simulink model "sim_real_data"  (R2022b)
settings: Solver=FixedStepAuto  StartTime=0.0  StopTime=15  FixedStep=0.002  RelTol=1e-3
undefined symbols (not defined in the file): c, c0, dT, k, k0
libraries: sharedTrackingLibrary x2, simulink x1
settings Model: Creator=lucabeber  LastModifiedBy=lucabeber

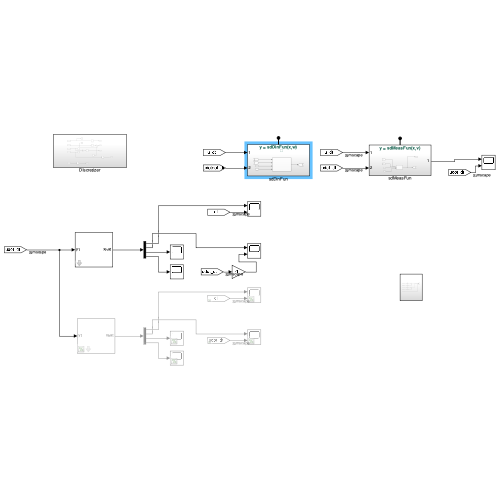
[thumbnail: Simulink's stored preview of the top-level diagram]
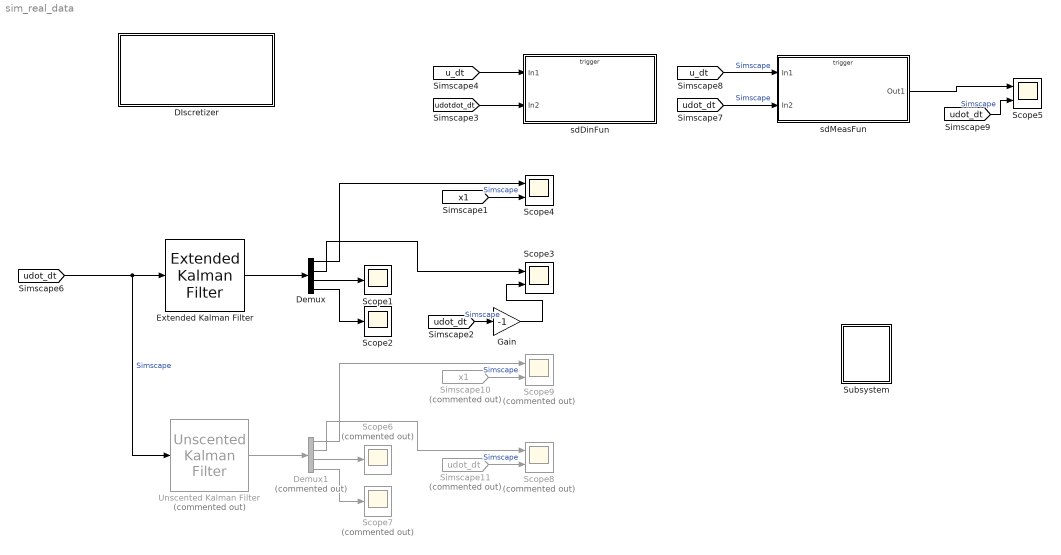
== system sim_real_data ==
  DIscretizer : Subsystem
  Demux : Demux
  Demux1 : Demux  Commented=on
  Extended Kalman Filter : sharedTrackingLibrary/Extended Kalman Filter  StateTransitionFcn=sdDinFun  HasStateTransitionJacobianFcn=off  HasAdditiveProcessNoise=Nonadditive  ProcessNoise=0  HasTimeVaryingProcessNoise=off  HasStateTransitionFcnExtraArgument=0  InitialState=[0,0,5e4,50]  InitialStateCovariance=[1,1,1e7,10]  MeasurementFcn1=sdMeasFun  HasMeasurementJacobianFcn1=off  HasMeasurementEnablePort1=off  HasAdditiveMeasurementNoise1=Nonadditive  MeasurementNoise1=0.00005  HasTimeVaryingMeasurementNoise1=off  HasMeasurementFcnExtraArgument1=0  HasMeasurementWrapping1=off  MeasurementFcn2=myMeasurementFcn  HasMeasurementJacobianFcn2=off  HasMeasurementEnablePort2=off  HasAdditiveMeasurementNoise2=Additive  MeasurementNoise2=1  HasTimeVaryingMeasurementNoise2=off  HasMeasurementFcnExtraArgument2=0  HasMeasurementWrapping2=off  MeasurementFcn3=myMeasurementFcn  HasMeasurementJacobianFcn3=off  HasMeasurementEnablePort3=off  HasAdditiveMeasurementNoise3=Additive  MeasurementNoise3=1  HasTimeVaryingMeasurementNoise3=off  HasMeasurementFcnExtraArgument3=0  HasMeasurementWrapping3=off  MeasurementFcn4=myMeasurementFcn  HasMeasurementJacobianFcn4=off  HasMeasurementEnablePort4=off  HasAdditiveMeasurementNoise4=Additive  MeasurementNoise4=1  HasTimeVaryingMeasurementNoise4=off  HasMeasurementFcnExtraArgument4=0  HasMeasurementWrapping4=off  MeasurementFcn5=myMeasurementFcn  HasMeasurementJacobianFcn5=off  HasMeasurementEnablePort5=off  HasAdditiveMeasurementNoise5=Additive  MeasurementNoise5=1  HasTimeVaryingMeasurementNoise5=off  HasMeasurementFcnExtraArgument5=0  HasMeasurementWrapping5=off  EnableMultirate=off  StateTransitionFcnSampleTime=1  MeasurementFcn1SampleTime=1  MeasurementFcn2SampleTime=1  MeasurementFcn3SampleTime=1  MeasurementFcn4SampleTime=1  MeasurementFcn5SampleTime=1  UseCurrentEstimator=on  OutputStateCovariance=off  DataType=double  SampleTime=dT  NumberOfMeasurements=1
  Gain : Gain  Gain=-1
  Scope1 : Scope
  Scope2 : Scope
  Scope3 : Scope  NumInputPorts=2
  Scope4 : Scope  NumInputPorts=2
  Scope5 : Scope  NumInputPorts=2
  Scope6 : Scope  Commented=on
  Scope7 : Scope  Commented=on
  Scope8 : Scope  Commented=on  NumInputPorts=2
  Scope9 : Scope  Commented=on  NumInputPorts=2
  Simscape10 : From  Commented=on  GotoTag=x1  TagVisibility=global
  Simscape11 : From  Commented=on  GotoTag=udot_dt  TagVisibility=global
  Subsystem : Subsystem
  Unscented Kalman Filter : sharedTrackingLibrary/Unscented Kalman Filter  Commented=on  StateTransitionFcn=sdDinFun  HasAdditiveProcessNoise=Nonadditive  ProcessNoise=0  HasTimeVaryingProcessNoise=off  HasStateTransitionFcnExtraArgument=0  InitialState=[0,0,1,1]  InitialStateCovariance=1  Alpha=1e-3  Beta=2  Kappa=0  MeasurementFcn1=sdMeasFun  HasMeasurementEnablePort1=off  HasAdditiveMeasurementNoise1=Nonadditive  MeasurementNoise1=0.01  HasTimeVaryingMeasurementNoise1=off  HasMeasurementFcnExtraArgument1=0  HasMeasurementWrapping1=off  MeasurementFcn2=myMeasurementFcn  HasMeasurementEnablePort2=off  HasAdditiveMeasurementNoise2=Additive  MeasurementNoise2=1  HasTimeVaryingMeasurementNoise2=off  HasMeasurementFcnExtraArgument2=0  HasMeasurementWrapping2=off  MeasurementFcn3=myMeasurementFcn  HasMeasurementEnablePort3=off  HasAdditiveMeasurementNoise3=Additive  MeasurementNoise3=1  HasTimeVaryingMeasurementNoise3=off  HasMeasurementFcnExtraArgument3=0  HasMeasurementWrapping3=off  MeasurementFcn4=myMeasurementFcn  HasMeasurementEnablePort4=off  HasAdditiveMeasurementNoise4=Additive  MeasurementNoise4=1  HasTimeVaryingMeasurementNoise4=off  HasMeasurementFcnExtraArgument4=0  HasMeasurementWrapping4=off  MeasurementFcn5=myMeasurementFcn  HasMeasurementEnablePort5=off  HasAdditiveMeasurementNoise5=Additive  MeasurementNoise5=1  HasTimeVaryingMeasurementNoise5=off  HasMeasurementFcnExtraArgument5=0  HasMeasurementWrapping5=off  EnableMultirate=off  StateTransitionFcnSampleTime=1  MeasurementFcn1SampleTime=1  MeasurementFcn2SampleTime=1  MeasurementFcn3SampleTime=1  MeasurementFcn4SampleTime=1  MeasurementFcn5SampleTime=1  UseCurrentEstimator=on  OutputStateCovariance=off  DataType=double  SampleTime=dT  NumberOfMeasurements=1
      settings: LibrarySourceBlock=cstblocks/State Estimation/Unscented Kalman Filter
  sdDinFun : Subsystem  TreatAsAtomicUnit=on
  sdMeasFun : Subsystem  TreatAsAtomicUnit=on
  wires:
  [udot_dt] -> Unscented Kalman Filter/1, Extended Kalman Filter/1  "Simscape"
  Extended Kalman Filter/1 -> Demux/1
  Demux/3 -> Scope1/1
  Demux/4 -> Scope2/1
  Demux/1 -> Scope4/1
  Demux/2 -> Scope3/1
  [x1] -> Scope4/2  "Simscape"
  [u_dt] -> sdDinFun/1(In1)
  [udotdot_dt] -> sdDinFun/2(In2)
  [u_dt] -> sdMeasFun/1(In1)  "Simscape"
  [udot_dt] -> sdMeasFun/2(In2)  "Simscape"
  sdMeasFun/1(Out1) -> Scope5/1
  [udot_dt] -> Scope5/2  "Simscape"
  Demux1/4 -> Scope7/1
  Demux1/1 -> Scope9/1
  Demux1/3 -> Scope6/1
  Simscape11/1 -> Scope8/2  "Simscape"
  Unscented Kalman Filter/1 -> Demux1/1
  Demux1/2 -> Scope8/1
  Simscape10/1 -> Scope9/2  "Simscape"
  [udot_dt] -> Gain/1  "Simscape"
  Gain/1 -> Scope3/2

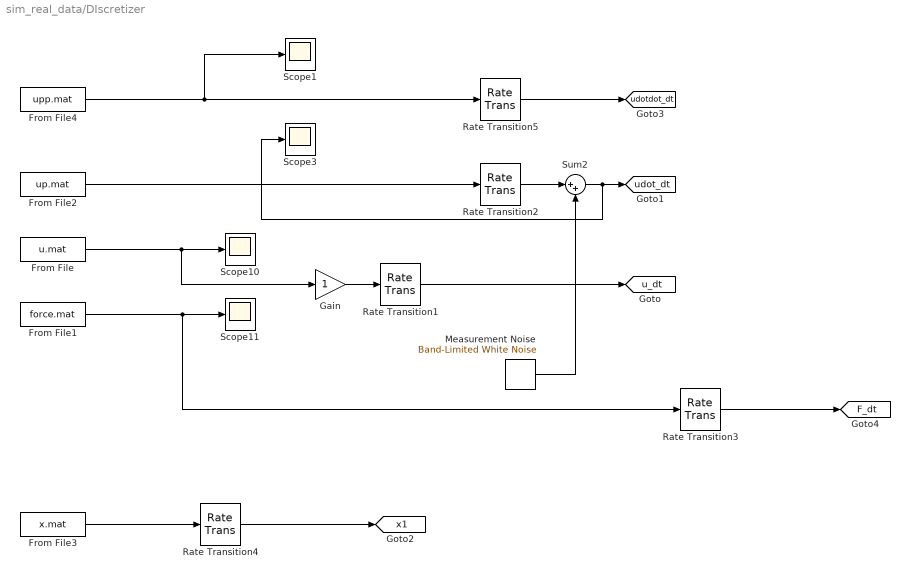
== system sim_real_data/DIscretizer ==
  From File : FromFile  FileName=u.mat  SampleTime=dT
  From File1 : FromFile  FileName=force.mat  SampleTime=dT
  From File2 : FromFile  FileName=up.mat  SampleTime=dT
  From File3 : FromFile  FileName=x.mat  SampleTime=dT
  From File4 : FromFile  FileName=upp.mat  SampleTime=dT
  Gain : Gain
  Measurement Noise : simulink/Sources/Band-Limited White Noise  Cov=1e-7  Ts=dT  seed=[23342]
  Rate Transition{1..5} (5 alike) : RateTransition  OutPortSampleTime=dT
  Scope{1,3,10..11} (4 alike) : Scope
  Sum2 : Sum  Inputs=|++
  tag scope: F_dt=global, u_dt=global, udot_dt=global, udotdot_dt=global, x1=global
  wires:
  Rate Transition3/1 -> [F_dt]
  From File/1 -> Gain/1, Scope10/1
  From File1/1 -> Rate Transition3/1, Scope11/1
  Rate Transition1/1 -> [u_dt]
  Rate Transition2/1 -> Sum2/1
  From File2/1 -> Rate Transition2/1
  From File3/1 -> Rate Transition4/1
  Rate Transition4/1 -> [x1]
  Gain/1 -> Rate Transition1/1
  Rate Transition5/1 -> [udotdot_dt]
  From File4/1 -> Scope1/1, Rate Transition5/1
  Measurement Noise/1 -> Sum2/2
  Sum2/1 -> Scope3/1, [udot_dt]

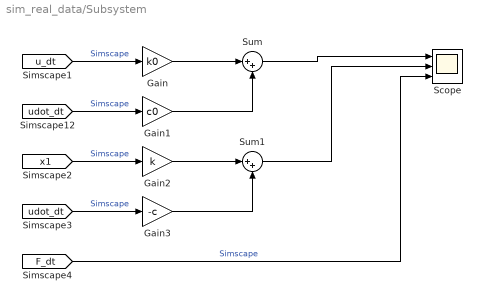
== system sim_real_data/Subsystem ==
  Gain : Gain  Gain=k0
  Gain1 : Gain  Gain=c0
  Gain2 : Gain  Gain=k
  Gain3 : Gain  Gain=-c
  Scope : Scope  NumInputPorts=3
  Sum : Sum  Inputs=|++
  Sum1 : Sum  Inputs=|++
  wires:
  [u_dt] -> Gain/1  "Simscape"
  Gain/1 -> Sum/1
  [udot_dt] -> Gain1/1  "Simscape"
  Gain1/1 -> Sum/2
  Sum/1 -> Scope/1
  [udot_dt] -> Gain3/1  "Simscape"
  Gain3/1 -> Sum1/2
  Sum1/1 -> Scope/2
  [x1] -> Gain2/1  "Simscape"
  Gain2/1 -> Sum1/1
  [F_dt] -> Scope/3  "Simscape"

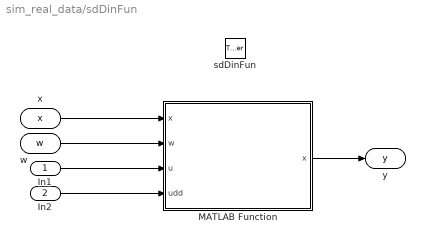
== system sim_real_data/sdDinFun ==
  In1 : Inport
  In2 : Inport  Port=2
  sdDinFun : TriggerPort  TriggerType=function-call  IsSimulinkFunction=on  FunctionName=sdDinFun  FunctionVisibility=scoped  VariantControl=(inherit)
  MATLAB Function : MATLAB Function  TreatAsAtomicUnit=on
  x : ArgIn  DisableCoverage=on  PortDimensions=4  ArgumentName=x
  w : ArgIn  DisableCoverage=on  Port=2  ArgumentName=w
  y : ArgOut  DisableCoverage=on  PortDimensions=4  ArgumentName=y
  wires:
  MATLAB Function/1(x) -> y/1
  x/1 -> MATLAB Function/1("x ")
  w/1 -> MATLAB Function/2(w)
  In1/1 -> MATLAB Function/3(u)
  In2/1 -> MATLAB Function/4(udd)

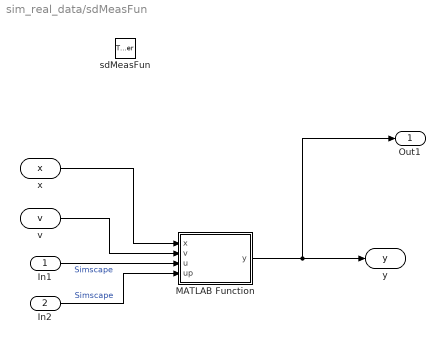
== system sim_real_data/sdMeasFun ==
  In1 : Inport
  In2 : Inport  Port=2
  sdMeasFun : TriggerPort  TriggerType=function-call  IsSimulinkFunction=on  FunctionName=sdMeasFun  FunctionVisibility=scoped  VariantControl=(inherit)
  MATLAB Function : MATLAB Function  TreatAsAtomicUnit=on
  x : ArgIn  DisableCoverage=on  PortDimensions=4  ArgumentName=x
  v : ArgIn  DisableCoverage=on  Port=2  ArgumentName=v
  y : ArgOut  DisableCoverage=on  ArgumentName=y
  Out1 : Outport  VectorParamsAs1DForOutWhenUnconnected=off
  wires:
  MATLAB Function/1(y) -> Out1/1, y/1
  x/1 -> MATLAB Function/1(x)
  v/1 -> MATLAB Function/2(v)
  In1/1 -> MATLAB Function/3(u)  "Simscape"
  In2/1 -> MATLAB Function/4(up)  "Simscape"

== matlab function sim_real_data/sdDinFun/MATLAB Function ==
  data: x input; x output; w input; u input; udd input
function x = sdDinFun(x,w,u,udd)
dT = 0.002; % s
m = 0.1; % kg
amp_disp = 0.01; % m
freq_disp = 5; % Hz
k0 = 200; % N/m
c0 = -8.8; % N/(m/s)
k = 1000; % N
c = 20; % N/(m/s) 
R1 = 0.03;  
m0 = 2.5;

% stiffness contribution
%sc = -  4/3 * (4 * x(3)) * x(1) * sqrt(2*R1*x(1));
%sc = -x(1)*x(3);
% damping constribution
%dc = - 2 * (4*x(4)) * sqrt(2*R1*x(1)) * x(2);
%dc = -x(2)*x(4);

x = [
    x(1) + dT * x(2);
    ( k0*(u) + m0 * udd - x(1)*x(3) )/( x(4) + c0 ) + w;
    x(3);
    x(4); 
];
% x = [
%     x(1) + dT * x(2);
%     ( k0*(u) - 4/3*(4*x(3))*x(1)*sqrt(abs(2*R1*x(1))) )/( 2*(4*x(4))*sqrt(abs(2*R1*x(1))) + c0) + w;
%     x(3);
%     x(4); 
% ];

== matlab function sim_real_data/sdMeasFun/MATLAB Function ==
  data: x input; y output; v input; u input; up input
function y = fnc(x,v,u,up)

dT = 1/(2e3); % s
m = 1; % kg
amp_disp = 0.01; % m
freq_disp = 5; % Hz
k0 = 200; % N/m
c0 = 20; % N/(m/s)
k = 1000; % N
c = 20; % N/(m/s)
%y = k0 * (-x(1) + u)+ c0 * (-x(2) + up) + v; %+ c0 * (-x(2) + up)  + v;
y = -x(2) + v;

end
